simulink model "lookup_nD_TestGen37"  (R2017b)
settings: Solver=FixedStepDiscrete  StartTime=0.0  StopTime=10.0  RelTol=1e-3
settings Model: Creator=ktrinh  LastModifiedBy=ktrinh
settings DebuggingCC: ParameterOverflowMsg=none

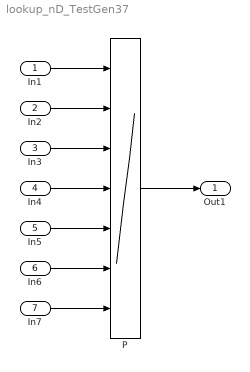
== system lookup_nD_TestGen37 ==
  In1 : Inport  OutMin=0  OutMax=127  OutDataTypeStr=uint8  PortDimensions=1
  In2 : Inport  Port=2  OutMin=0  OutMax=127  OutDataTypeStr=uint8
  In3 : Inport  Port=3  OutMin=0  OutMax=127  OutDataTypeStr=uint8
  In4 : Inport  Port=4  OutMin=0  OutMax=127  OutDataTypeStr=uint8
  In5 : Inport  Port=5  OutMin=0  OutMax=127  OutDataTypeStr=uint8
  In6 : Inport  Port=6  OutMin=0  OutMax=127  OutDataTypeStr=uint8
  In7 : Inport  Port=7  OutMin=0  OutMax=127  OutDataTypeStr=uint8
  P : Lookup_n-D  NumberOfTableDimensions=7  BreakpointsForDimension1=[20.6449487081805;28.9590977599481]  BreakpointsForDimension2=[2.79782437003312;21.1955109695439;29.5424297546603;45.7497711838768;64.6612064780801]  BreakpointsForDimension3=[12.6489991545786;17.3744968876799;45.0944426845204]  BreakpointsForDimension4=[5.41023020843354;49.7712491403735]  BreakpointsForDimension5=[90.1555615293621;93.1167458708717;98.1130419104113]  BreakpointsForDimension6=[2.49538002813475;23.506191693022;65.5266092442601;82.3934750598976]  BreakpointsForDimension7=[1.8469883161188;35.121342952892;79.1136962846033]  BreakpointsForDimension1DataTypeStr=uint16  BreakpointsForDimension2DataTypeStr=uint16  BreakpointsForDimension3DataTypeStr=uint16  BreakpointsForDimension4DataTypeStr=uint16  BreakpointsForDimension5DataTypeStr=uint16  BreakpointsForDimension6DataTypeStr=uint16  BreakpointsForDimension7DataTypeStr=uint16  Table=reshape(repmat([4 5 6 7 8;16 19 20 21 22;10 18 23 24 25],18,8),[2,5,3,2,3,4,3])  TableDataTypeStr=single  InterpMethod=Flat  ExtrapMethod=Clip  InternalRulePriority=Speed  OutDataTypeStr=uint16  SaturateOnIntegerOverflow=on  InputSameDT=on
  Out1 : Outport
  wires:
  In1/1 -> P/1
  In2/1 -> P/2
  In3/1 -> P/3
  In4/1 -> P/4
  In5/1 -> P/5
  In6/1 -> P/6
  In7/1 -> P/7
  P/1 -> Out1/1
